simulink model "giacc_ut"  (Simulink 8.1)
settings: Solver=FixedStepDiscrete  StartTime=0.0  StopTime=Inf  FixedStep=0.005  RelTol=1e-3
libraries: siltestlib x10, idiada_lib x4, giacc x1
settings Model: Creator=xsellart  LastModifiedBy=AT015555
settings DataIOCC: SignalLoggingSaveFormat=Dataset
settings OptimizationCC: ExpressionDepthLimit=128
settings DebuggingCC: FcnCallInpInsideContextMsg=EnableAllAsError
settings GRTTargetCC: CombineOutputUpdateFcns=on  GRTInterface=off

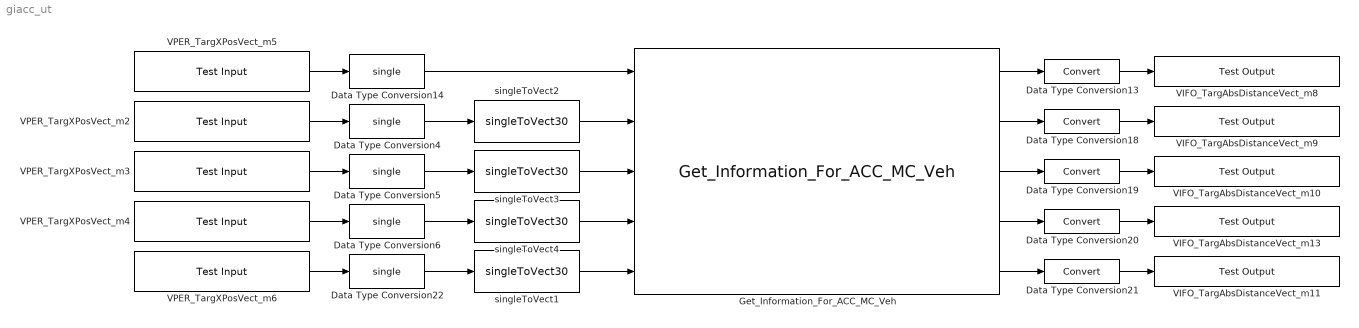
== system giacc_ut ==
  Data Type Conversion{13,18..21} (5 alike) : DataTypeConversion
  Data Type Conversion{4..6,14,22} (5 alike) : DataTypeConversion  OutDataTypeStr=single
  Get_Information_For_ACC_MC_Veh : giacc/Get_Information_For_ACC_MC_Veh
  VIFO_TargAbsDistanceVect_m10 : siltestlib/Test Output  varname=NIFO_ACCTargetVehAssigned_flg  sampletime=-1
  VIFO_TargAbsDistanceVect_m11 : siltestlib/Test Output  varname=NIFO_ACCMCLongAccel_mps2  sampletime=-1
  VIFO_TargAbsDistanceVect_m13 : siltestlib/Test Output  varname=NIFO_ACCMCVehId_num  sampletime=-1
  VIFO_TargAbsDistanceVect_m8 : siltestlib/Test Output  varname=NIFO_ACCTargetVehRelSpeedX_mps  sampletime=-1
  VIFO_TargAbsDistanceVect_m9 : siltestlib/Test Output  varname=NIFO_ACCMCVehXPosition_m  sampletime=-1
  VPER_TargXPosVect_m2 : siltestlib/Test Input  varname=VPER_TargXPosVect30_m  sampletime=0.005
  VPER_TargXPosVect_m3 : siltestlib/Test Input  varname=VIFO_TargVehRelSpdXVect30_mps  sampletime=0.005
  VPER_TargXPosVect_m4 : siltestlib/Test Input  varname=VPER_TargIdVect30_num  sampletime=0.005
  VPER_TargXPosVect_m5 : siltestlib/Test Input  varname=VIFO_ACCMCTTargetId_num  sampletime=0.005
  VPER_TargXPosVect_m6 : siltestlib/Test Input  varname=VIFO_TargAccelXVect30_mps2  sampletime=0.005
  singleToVect{1..4} (4 alike) : idiada_lib/singleToVect30
  wires:
  VPER_TargXPosVect_m2/1 -> Data Type Conversion4/1
  Data Type Conversion4/1 -> singleToVect2/1
  VPER_TargXPosVect_m3/1 -> Data Type Conversion5/1
  Data Type Conversion5/1 -> singleToVect3/1
  VPER_TargXPosVect_m4/1 -> Data Type Conversion6/1
  Data Type Conversion6/1 -> singleToVect4/1
  Data Type Conversion13/1 -> VIFO_TargAbsDistanceVect_m8/1
  singleToVect2/1 -> Get_Information_For_ACC_MC_Veh/2
  singleToVect3/1 -> Get_Information_For_ACC_MC_Veh/3
  singleToVect4/1 -> Get_Information_For_ACC_MC_Veh/4
  VPER_TargXPosVect_m5/1 -> Data Type Conversion14/1
  Data Type Conversion14/1 -> Get_Information_For_ACC_MC_Veh/1
  Get_Information_For_ACC_MC_Veh/1 -> Data Type Conversion13/1
  Data Type Conversion18/1 -> VIFO_TargAbsDistanceVect_m9/1
  Get_Information_For_ACC_MC_Veh/2 -> Data Type Conversion18/1
  Data Type Conversion19/1 -> VIFO_TargAbsDistanceVect_m10/1
  Get_Information_For_ACC_MC_Veh/3 -> Data Type Conversion19/1
  Data Type Conversion20/1 -> VIFO_TargAbsDistanceVect_m13/1
  Get_Information_For_ACC_MC_Veh/4 -> Data Type Conversion20/1
  Data Type Conversion21/1 -> VIFO_TargAbsDistanceVect_m11/1
  Get_Information_For_ACC_MC_Veh/5 -> Data Type Conversion21/1
  VPER_TargXPosVect_m6/1 -> Data Type Conversion22/1
  Data Type Conversion22/1 -> singleToVect1/1
  singleToVect1/1 -> Get_Information_For_ACC_MC_Veh/5
